simulink model "tema8"  (R2023b)
settings: Solver=VariableStepAuto  StartTime=0.0  StopTime=50  RelTol=1e-3
values from neighbouring files (symbols this model uses):
  k = 1.5    [tema8_m.m]
settings Model: Creator=chapo  LastModifiedBy=chapo

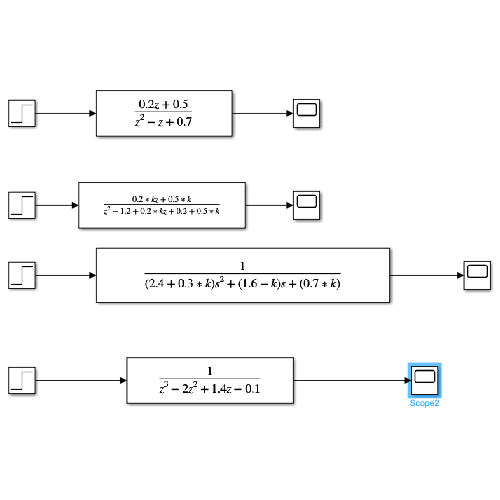
[thumbnail: Simulink's stored preview of the top-level diagram]
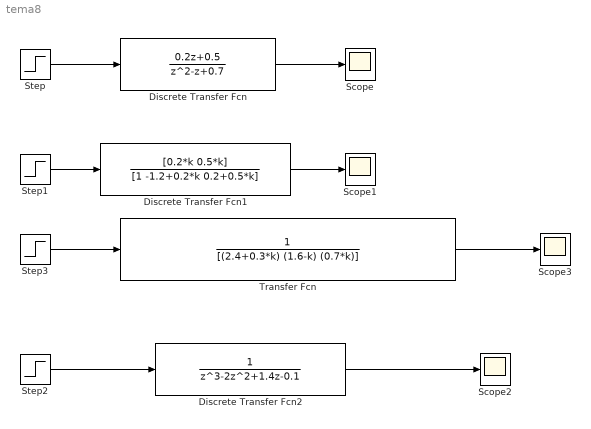
== system tema8 ==
  Discrete Transfer Fcn : DiscreteTransferFcn  Numerator=[0.2 0.5]  Denominator=[1 -1 0.7]  SampleTime=0.05
  Discrete Transfer Fcn1 : DiscreteTransferFcn  Numerator=[0.2*k 0.5*k]  Denominator=[1 -1.2+0.2*k 0.2+0.5*k]  SampleTime=0.05
  Discrete Transfer Fcn2 : DiscreteTransferFcn  Denominator=[1 -2 1.4 -0.1]  SampleTime=0.05
  Scope{,1..3} (4 alike) : Scope
  Step{,1..3} (4 alike) : Step  SampleTime=0
  Transfer Fcn : TransferFcn  Denominator=[(2.4+0.3*k) (1.6-k) (0.7*k)]
  wires:
  Step/1 -> Discrete Transfer Fcn/1
  Discrete Transfer Fcn/1 -> Scope/1
  Step1/1 -> Discrete Transfer Fcn1/1
  Discrete Transfer Fcn1/1 -> Scope1/1
  Discrete Transfer Fcn2/1 -> Scope2/1
  Step3/1 -> Transfer Fcn/1
  Transfer Fcn/1 -> Scope3/1
  Step2/1 -> Discrete Transfer Fcn2/1
